simulink model "scen1_BSCproposed"  (R2021b)
settings: Solver=ode4  StartTime=0.0  StopTime=tsim  FixedStep=sampleRate  RelTol=1e-3
undefined symbols (not defined in the file): des_z, Kb, Kbz, peak_mp, Q, saturation_on, t_end_mp
libraries: dspmtrx3 x1
settings Model: Creator=PC  LastModifiedBy=kangm
settings SolverCC: AlgebraicLoopSolver=TrustRegion
settings DataIOCC: ReturnWorkspaceOutputs=off
settings DebuggingCC: SFMachineParentedDataDiag=warning

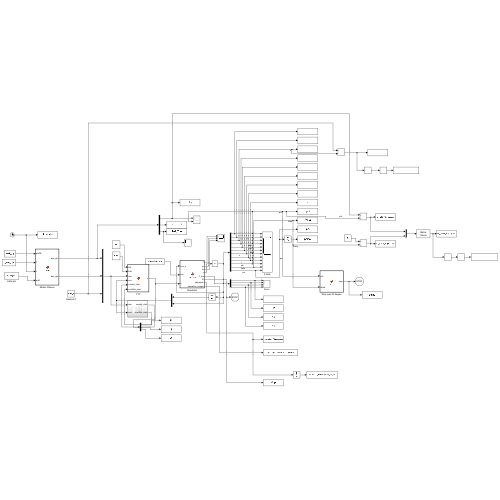
[thumbnail: Simulink's stored preview of the top-level diagram]
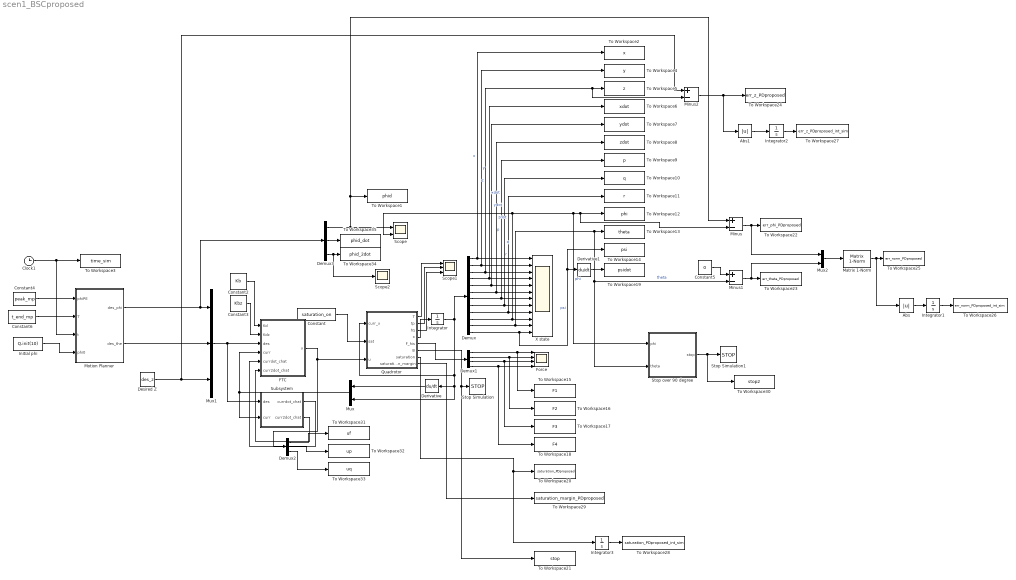
== system scen1_BSCproposed ==
  Abs : Abs
  Abs1 : Abs
  Clock1 : Clock
  Constant : Constant  Value=saturation_on
  Constant2 : Constant  Value=Kb
  Constant3 : Constant  Value=Kbz
  Constant4 : Constant  Value=peak_mp
  Constant5 : Constant  Value=0
  Constant6 : Constant  Value=t_end_mp
  Demux : Demux  Outputs=12
  Demux1 : Demux
  Demux2 : Demux  Outputs=3
  Demux3 : Demux  Outputs=3
  Derivative : Derivative
  Derivative1 : Derivative
  Desired Z : Constant  Value=des_z
  FTC : MATLAB Function  TreatAsAtomicUnit=on
  Force : Scope  NumInputPorts=4
  Initial phi : Constant  Value=Q.init(10)
  Integrator : Integrator  InitialCondition=Q.init
  Integrator1 : Integrator
  Integrator2 : Integrator
  Integrator3 : Integrator
  Matrix 1-Norm : dspmtrx3/Matrix  1-Norm  roundingMode=Floor  overflowMode=off  outputDataTypeStr=Inherit: Same as accumulator  outputMin=[]  outputMax=[]  outputLastDataTypeStr=Inherit: Same as accumulator
      settings: SourceProductBaseCode=DS
  Minus : Sum  Inputs=+-
  Minus1 : Sum  Inputs=+-
  Minus2 : Sum  Inputs=+-
  Motion Planner : MATLAB Function  TreatAsAtomicUnit=on
  Mux : Mux  Inputs=2
  Mux1 : Mux  Inputs=3
  Mux2 : Mux  Inputs=2
  Quadrotor : MATLAB Function  TreatAsAtomicUnit=on
  Scope : Scope  NumInputPorts=2
  Scope1 : Scope  NumInputPorts=3
  Scope2 : Scope
  Stop Simulation : Stop
  Stop Simulation1 : Stop
  Stop over 90 degree : MATLAB Function  TreatAsAtomicUnit=on
  Subsystem : Subsystem
  To Workspace1 : ToWorkspace  VariableName=phid  SampleTime=-1
      settings: Save2DSignal=2-D array (concatenate along first dimension)
  To Workspace10 : ToWorkspace  VariableName=q  SampleTime=-1
      settings: Save2DSignal=2-D array (concatenate along first dimension)
  To Workspace11 : ToWorkspace  VariableName=r  SampleTime=-1
      settings: Save2DSignal=2-D array (concatenate along first dimension)
  To Workspace12 : ToWorkspace  VariableName=phi  SampleTime=-1
      settings: Save2DSignal=2-D array (concatenate along first dimension)
  To Workspace13 : ToWorkspace  VariableName=theta  SampleTime=-1
      settings: Save2DSignal=2-D array (concatenate along first dimension)
  To Workspace14 : ToWorkspace  VariableName=psi  SampleTime=-1
      settings: Save2DSignal=2-D array (concatenate along first dimension)
  To Workspace15 : ToWorkspace  VariableName=F1  SampleTime=-1
      settings: Save2DSignal=2-D array (concatenate along first dimension)
  To Workspace16 : ToWorkspace  VariableName=F2  SampleTime=-1
      settings: Save2DSignal=2-D array (concatenate along first dimension)
  To Workspace17 : ToWorkspace  VariableName=F3  SampleTime=-1
      settings: Save2DSignal=2-D array (concatenate along first dimension)
  To Workspace18 : ToWorkspace  VariableName=F4  SampleTime=-1
      settings: Save2DSignal=2-D array (concatenate along first dimension)
  To Workspace19 : ToWorkspace  VariableName=psidot  SampleTime=-1
      settings: Save2DSignal=2-D array (concatenate along first dimension)
  To Workspace2 : ToWorkspace  VariableName=x  SampleTime=-1
      settings: Save2DSignal=2-D array (concatenate along first dimension)
  To Workspace20 : ToWorkspace  VariableName=saturation_PDproposed  SampleTime=-1
      settings: Save2DSignal=2-D array (concatenate along first dimension)
  To Workspace21 : ToWorkspace  VariableName=stop  SampleTime=-1
      settings: Save2DSignal=2-D array (concatenate along first dimension)
  To Workspace22 : ToWorkspace  VariableName=err_phi_PDproposed  SampleTime=-1
      settings: Save2DSignal=2-D array (concatenate along first dimension)
  To Workspace23 : ToWorkspace  VariableName=err_theta_PDproposed  SampleTime=-1
      settings: Save2DSignal=2-D array (concatenate along first dimension)
  To Workspace24 : ToWorkspace  VariableName=err_z_PDproposed  SampleTime=-1
      settings: Save2DSignal=2-D array (concatenate along first dimension)
  To Workspace25 : ToWorkspace  VariableName=err_norm_PDproposed  SampleTime=-1
      settings: Save2DSignal=2-D array (concatenate along first dimension)
  To Workspace26 : ToWorkspace  VariableName=err_norm_PDproposed_int_sim  SampleTime=-1
      settings: Save2DSignal=2-D array (concatenate along first dimension)
  To Workspace27 : ToWorkspace  VariableName=err_z_PDproposed_int_sim  SampleTime=-1
      settings: Save2DSignal=2-D array (concatenate along first dimension)
  To Workspace28 : ToWorkspace  VariableName=saturation_PDproposed_int_sim  SampleTime=-1
      settings: Save2DSignal=2-D array (concatenate along first dimension)
  To Workspace29 : ToWorkspace  VariableName=saturation_margin_PDproposed  SampleTime=-1
      settings: Save2DSignal=2-D array (concatenate along first dimension)
  To Workspace3 : ToWorkspace  VariableName=time_sim  SampleTime=-1
      settings: Save2DSignal=2-D array (concatenate along first dimension)
  To Workspace30 : ToWorkspace  VariableName=stop2  SampleTime=-1
      settings: Save2DSignal=2-D array (concatenate along first dimension)
  To Workspace31 : ToWorkspace  VariableName=uf  SampleTime=-1
      settings: Save2DSignal=2-D array (concatenate along first dimension)
  To Workspace32 : ToWorkspace  VariableName=up  SampleTime=-1
      settings: Save2DSignal=2-D array (concatenate along first dimension)
  To Workspace33 : ToWorkspace  VariableName=uq  SampleTime=-1
      settings: Save2DSignal=2-D array (concatenate along first dimension)
  To Workspace34 : ToWorkspace  VariableName=phid_2dot  SampleTime=-1
      settings: Save2DSignal=2-D array (concatenate along first dimension)
  To Workspace35 : ToWorkspace  VariableName=phid_dot  SampleTime=-1
      settings: Save2DSignal=2-D array (concatenate along first dimension)
  To Workspace4 : ToWorkspace  VariableName=y  SampleTime=-1
      settings: Save2DSignal=2-D array (concatenate along first dimension)
  To Workspace5 : ToWorkspace  VariableName=z  SampleTime=-1
      settings: Save2DSignal=2-D array (concatenate along first dimension)
  To Workspace6 : ToWorkspace  VariableName=xdot  SampleTime=-1
      settings: Save2DSignal=2-D array (concatenate along first dimension)
  To Workspace7 : ToWorkspace  VariableName=ydot  SampleTime=-1
      settings: Save2DSignal=2-D array (concatenate along first dimension)
  To Workspace8 : ToWorkspace  VariableName=zdot  SampleTime=-1
      settings: Save2DSignal=2-D array (concatenate along first dimension)
  To Workspace9 : ToWorkspace  VariableName=p  SampleTime=-1
      settings: Save2DSignal=2-D array (concatenate along first dimension)
  X state : Scope  NumInputPorts=12
  wires:
  Quadrotor/4(x) -> Integrator/1
  Mux1/1 -> Subsystem/1(des), FTC/3(des)
  Integrator/1 -> Quadrotor/1(curr_x), Derivative/1, Mux/2, Demux/1
  Demux/1 -> To Workspace2/1, X state/1  "x"
  Demux/2 -> To Workspace4/1, X state/2  "y"
  Demux/4 -> To Workspace6/1, X state/4  "xdot"
  Demux/5 -> To Workspace7/1, X state/5  "ydot"
  Demux/6 -> To Workspace8/1, X state/6  "zdot"
  Demux/7 -> To Workspace9/1, X state/7  "p"
  Demux/8 -> To Workspace10/1, X state/8  "q"
  Demux/9 -> To Workspace11/1, X state/9  "r"
  Mux/1 -> FTC/4(curr), Subsystem/2(curr)
  Derivative/1 -> Mux/1
  Quadrotor/5(F_his) -> Demux1/1
  Demux1/1 -> To Workspace15/1, Force/1
  Demux1/3 -> To Workspace17/1, Force/3
  Demux1/4 -> To Workspace18/1, Force/4
  Demux1/2 -> Force/2, To Workspace16/1
  Demux/12 -> To Workspace14/1, Derivative1/1, X state/12  "psi"
  Derivative1/1 -> To Workspace19/1
  Demux3/1 -> To Workspace1/1, Minus/1, Scope/1
  Constant/1 -> Quadrotor/2(sat)
  Clock1/1 -> Motion Planner/3(t), To Workspace3/1
  Initial phi/1 -> Motion Planner/4(phi0)
  Demux3/2 -> To Workspace35/1
  Demux3/3 -> Scope2/1, To Workspace34/1
  FTC/1(u) -> Demux2/1, Quadrotor/3(u)
  Quadrotor/1(T) -> Scope1/1
  Quadrotor/3(tq) -> Scope1/3
  Quadrotor/2(tp) -> Scope1/2
  Motion Planner/1(des_phi) -> Demux3/1, Mux1/1
  Motion Planner/2(des_the) -> Mux1/2
  Quadrotor/6(B) -> To Workspace21/1, Stop Simulation/1
  Desired Z/1 -> Minus2/1, Mux1/3
  Minus1/1 -> Mux2/2, To Workspace23/1
  Minus/1 -> Mux2/1, To Workspace22/1
  Demux/3 -> Minus2/2, To Workspace5/1, X state/3  "z"
  Mux2/1 -> Matrix 1-Norm/1
  Constant5/1 -> Minus1/1
  Integrator1/1 -> To Workspace26/1
  Matrix 1-Norm/1 -> Abs/1, To Workspace25/1
  Abs/1 -> Integrator1/1
  Constant4/1 -> Motion Planner/1(phiPE)
  Constant6/1 -> Motion Planner/2(T)
  Integrator2/1 -> To Workspace27/1
  Minus2/1 -> Abs1/1, To Workspace24/1
  Abs1/1 -> Integrator2/1
  Integrator3/1 -> To Workspace28/1
  Quadrotor/7(saturation) -> Integrator3/1, To Workspace20/1
  Quadrotor/8(saturation_margin) -> To Workspace29/1
  Demux/10 -> Scope/2, Stop over 90 degree/1(phi), Minus/2, To Workspace12/1, X state/10  "phi"
  Stop over 90 degree/1(stop) -> To Workspace30/1, Stop Simulation1/1
  Demux/11 -> Stop over 90 degree/2(theta), Minus1/2, To Workspace13/1, X state/11  "theta"
  Demux2/1 -> To Workspace31/1
  Demux2/2 -> To Workspace32/1
  Demux2/3 -> To Workspace33/1
  Constant2/1 -> FTC/1(Kd)
  Subsystem/1(currdot_chat) -> FTC/5(currdot_chat)
  Subsystem/2(curr2dot_chat) -> FTC/6(curr2dot_chat)
  Constant3/1 -> FTC/2(Kdz)

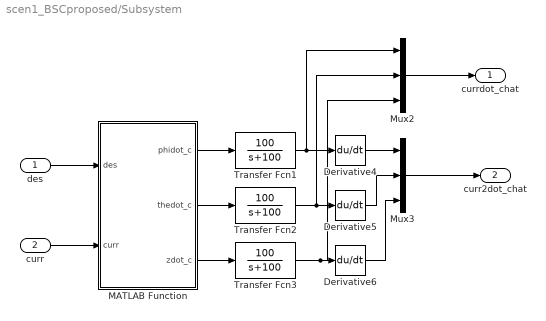
== system scen1_BSCproposed/Subsystem ==
  des : Inport
  curr : Inport  Port=2
  Derivative4 : Derivative
  Derivative5 : Derivative
  Derivative6 : Derivative
  MATLAB Function : MATLAB Function  TreatAsAtomicUnit=on
  Mux2 : Mux  Inputs=3
  Mux3 : Mux  Inputs=3
  Transfer Fcn1 : TransferFcn  Numerator=[100]  Denominator=[1 100]
  Transfer Fcn2 : TransferFcn  Numerator=[100]  Denominator=[1 100]
  Transfer Fcn3 : TransferFcn  Numerator=[100]  Denominator=[1 100]
  currdot_chat : Outport
  curr2dot_chat : Outport  Port=2
  wires:
  Derivative6/1 -> Mux3/3
  des/1 -> MATLAB Function/1(des)
  MATLAB Function/3(zdot_c) -> Transfer Fcn3/1
  Transfer Fcn2/1 -> Mux2/2, Derivative5/1
  MATLAB Function/1(phidot_c) -> Transfer Fcn1/1
  MATLAB Function/2(thedot_c) -> Transfer Fcn2/1
  Transfer Fcn3/1 -> Mux2/3, Derivative6/1
  Derivative4/1 -> Mux3/1
  Derivative5/1 -> Mux3/2
  Transfer Fcn1/1 -> Mux2/1, Derivative4/1
  Mux2/1 -> currdot_chat/1
  Mux3/1 -> curr2dot_chat/1
  curr/1 -> MATLAB Function/2(curr)

== matlab function scen1_BSCproposed/Quadrotor ==
  data: T output; tp output; tq output; curr_x input; sat input; u input; x output; F_his output; B output; saturation output; saturation_margin output
function [T,tp,tq,x,F_his,B,saturation,saturation_margin] = system(curr_x,sat,u)
% x = {xyz xyzvel pqr phi theta psi}
x = zeros(12,1);
% Properties
m = 1.282; g = 9.81;
Ix = 4.856*10^-3; Iz = 8.801*10^-3;
b = 0.0066;
kr = 0.02; %drag coefficient
kt = 0.5;
l = 0.1;

u_temp = zeros(3,1);
u_temp = u;
u = u_temp;

T = u(1); tp = u(2); tq = u(3);% tr = u(4);
tr = b*(T-2*tp/l);
A = [1 1 1; 0 l 0;-l 0 l];

F=inv(A)*[T tp tq]';

f1 = F(1); f2 = F(2); f3 = F(3);
ub = 8.38;
lb = 0;

saturation1_lb = 0;
saturation1_ub = 0;
saturation2_lb = 0;
saturation2_ub = 0;
saturation3_lb = 0;
saturation3_ub = 0;
saturation1_lb_margin = 0;
saturation1_ub_margin = 0;
saturation2_lb_margin = 0;
saturation2_ub_margin = 0;
saturation3_lb_margin = 0;
saturation3_ub_margin = 0;

if sat == 1
    if f1 < lb
        saturation1_lb = abs(lb - f1);
        saturation1_lb_margin = abs(lb - f1);
        f1 = lb;
    else
        saturation1_lb_margin = lb - f1;
    end
    
    if f1 > ub
        saturation1_ub = abs(ub - f1);
        saturation1_ub_margin = abs(ub - f1);
        f1 = ub;
    else
        saturation1_ub_margin = f1 - ub;
    end
    
    if f2 < lb
        saturation2_lb = abs(lb - f2);
        saturation2_lb_margin = abs(lb - f2);
        f2 = lb;
    else
        saturation2_lb_margin = lb - f2;
    end
    
    if f2 > ub
        saturation2_ub = abs(ub - f2);
        saturation2_ub_margin = abs(ub - f2);
        f2 = ub;
    else
        saturation2_ub_margin = f2 - ub;
    end
    
    if f3 < lb
        saturation3_lb = abs(lb - f3);
        saturation3_lb_margin = abs(lb - f3);
        f3 = lb;
    else
        saturation3_lb_margin = lb - f3;
    end
    
    if f3 > ub
        saturation3_ub = abs(ub - f3);
        saturation3_ub_margin = abs(ub - f3);
        f3 = ub;
    else
        saturation3_ub_margin = f3 - ub;
    end
end

saturation = max([saturation1_lb,saturation1_ub,saturation2_lb,saturation2_ub,saturation3_lb,saturation3_ub]);
saturation_margin = max([saturation1_lb_margin,saturation1_ub_margin,saturation2_lb_margin,saturation2_ub_margin,saturation3_lb_margin,saturation3_ub_margin]);

f4 = 0;
F_his = [f1 f2 f3 f4]';
T = f1+f2+f3;
tp = l*(f2);
tq = l*(f3-f1);
tr = b*(f1+f3-f2);


% Current state
x1  = curr_x(1);
x2  = curr_x(2);
x3  = curr_x(3);
x4  = curr_x(4);
x5  = curr_x(5);
x6  = curr_x(6);
x7  = curr_x(7);
x8  = curr_x(8);
x9  = curr_x(9);
x10 = curr_x(10);
x11 = curr_x(11);
x12 = curr_x(12);


% Position
x(1) = x4;
x(2) = x5;
x(3) = x6;
% Velocity
x(4) = T/m*(cos(x12)*sin(x11)*cos(x10) + sin(x12)*sin(x10)) - kt/m*x4;
x(5) = T/m*(sin(x12)*sin(x11)*cos(x10) - cos(x12)*sin(x10)) - kt/m*x5;
x(6) = -g + T*(1/m)*(cos(x10)*cos(x11)) - kt/m*x6;
% Body rate
x(7) = ((Ix-Iz)*x8*x9 + tp)/Ix;
x(8) = ((Iz-Ix)*x7*x9 + tq)/Ix;
x(9) = (-kr*x9 + tr)/Iz;
% Angle
x(10) = x7 + x8*sin(x10)*tan(x11) + x9*cos(x10)*tan(x11);
x(11) = x8*cos(x10) - x9*sin(x10);
x(12) = x8*sin(x10)/cos(x11) + x9*cos(x10)*cos(x11);

if x3<=0
    B=1;
else
    B=0;
end

% x;
% 
% r_c = 10.2020-2.2725*x9;
% u_c = (x(7)-((Ix-Iz)/Ix)*x8*x9)*Ix+x10;
% r_ct = -4.489*exp(-2.2725*t)+4.489;

== matlab function scen1_BSCproposed/Stop over 90 degree ==
  data: phi input; stop output; theta input
function stop = fcn(phi, theta)

stop = 0;
max_attitude = deg2rad(90);

if abs(phi) >= max_attitude || abs(theta) >= max_attitude
    stop = 1;
end

== matlab function scen1_BSCproposed/Motion Planner ==
  data: phiPE input; T input; des_phi output; des_the output; t input; phi0 input
function [des_phi,des_the]  = fcn(phiPE,T,t,phi0)


% b = deg2rad(20); % Periodic solution phi
% t_end = 5;
a0 = phi0;
a1 = 0;
a2 = 0;
a3 = - (10*phi0 - 10*phiPE)/T^3;
a4 = (15*phi0 - 15*phiPE)/T^4;
a5 = -(6*phi0 - 6*phiPE)/T^5;

if t <= T
    phi_d = a0 + a1*t + a2*t^2 + a3*t^3 + a4*t^4 + a5*t^5; % phi_d(0) = phi(0) and phi_d(t_end) = phi hat (periodic solution)
    phidot_d = a1 + 2*a2*t + 3*a3*t^2 + 4*a4*t^3 + 5*a5*t^4; % phidot_d(t_end) = 0
    phi2dot_d = 2*a2 + 6*a3*t + 12*a4*t^2 + 20*a5*t^3;
else
    phi_d = phiPE;
    phidot_d = 0;
    phi2dot_d = 0;
end

% phidot_d = 0;

the_d = deg2rad(0); thedot_d = 0; the2dot_d = 0;


des_phi = [phi_d, phidot_d, phi2dot_d]';
des_the = [the_d, thedot_d, the2dot_d]';

== matlab function scen1_BSCproposed/FTC ==
  data: Kd input; Kdz input; des input; u output; curr input; currdot_chat input; curr2dot_chat input
function u   = bsc(Kd,Kdz,des,curr,currdot_chat,curr2dot_chat)

m = 1.282; g = 9.81;
Ix = 4.856*10^-3; Iy = Ix; Iz = 8.801*10^-3;
b = 0.0066;
kr = 0.02; %drag coefficient
kt = 0.5;
% kt = 0.25;
l = 0.1;

% current state
N = 0;
xdot   = curr(N+1); ydot   = curr(N+2); zdot   = curr(N+3);
x2dot  = curr(N+4); y2dot  = curr(N+5); z2dot  = curr(N+6);
pdot   = curr(N+7); qdot   = curr(N+8); rdot   = curr(N+9);
phidot = curr(N+10);thedot = curr(N+11);psidot = curr(N+12);

N = 12;
x    = curr(N+1); y    = curr(N+2); z    = curr(N+3);
xdot = curr(N+4); ydot = curr(N+5); zdot = curr(N+6);
p    = curr(N+7); q    = curr(N+8); r    = curr(N+9);
phi  = curr(N+10);the  = curr(N+11);psi  = curr(N+12);
des_temp = zeros(7,1);
des_temp = des;
des = des_temp;
% desired state
phi_d = des(1);
phidot_d = des(2);
phi2dot_d = des(3);
the_d = des(4);
thedot_d = des(5);
the2dot_d = des(6);
z_d   = des(7);

phidot_chat = currdot_chat(1);
thedot_chat = currdot_chat(2);
zdot_chat = currdot_chat(3);
phi2dot_chat = curr2dot_chat(1);
the2dot_chat = curr2dot_chat(2);
z2dot_chat = curr2dot_chat(3);

F = [p + q*sin(phi)*tan(the) + r*cos(phi)*tan(the)
     q*cos(phi) - r*sin(phi)
     -(Iz - Iy)*q*r/Ix
     -(Ix - Iz)*p*r/Iy
     -kr*r/Iz
     zdot
     -kt*zdot/m - g];
 
G = [0 0 0
     0 0 0
     0 1/Ix 0
     0 0 1/Iy
     b/Iz -2*b/(l*Iz) 0
     0 0 0
     cos(phi)*cos(the)/m 0 0];
 
J = [q*cos(phi)*tan(the)-r*sin(phi)*tan(the) q*sin(phi)*sec(the)^2+r*cos(phi)*sec(the)^2 1 sin(phi)*tan(the) cos(phi)*tan(the) 0 0
     -q*sin(phi)-r*cos(phi) 0 0 cos(phi) -sin(phi) 0 0
     0 0 0 0 0 0 1];

ubar = [phi2dot_chat + (phi_d-phi) + Kd*(phidot_chat-phidot)
        the2dot_chat + (the_d-the) + Kd*(thedot_chat-thedot)
        z2dot_chat + (0-zdot) + Kdz*(zdot_chat-zdot)];
    
u = inv(J*G)*(-J*F + ubar);

== matlab function scen1_BSCproposed/Subsystem/MATLAB Function ==
  data: des input; phidot_c output; curr input; thedot_c output; zdot_c output
function [phidot_c,thedot_c,zdot_c] = fcn(des, curr)

% current state
N = 0;
xdot   = curr(N+1); ydot   = curr(N+2); zdot   = curr(N+3);
x2dot  = curr(N+4); y2dot  = curr(N+5); z2dot  = curr(N+6);
pdot   = curr(N+7); qdot   = curr(N+8); rdot   = curr(N+9);
phidot = curr(N+10);thedot = curr(N+11);psidot = curr(N+12);

N = 12;
x    = curr(N+1); y    = curr(N+2); z    = curr(N+3);
xdot = curr(N+4); ydot = curr(N+5); zdot = curr(N+6);
p    = curr(N+7); q    = curr(N+8); r    = curr(N+9);
phi  = curr(N+10);the  = curr(N+11);psi  = curr(N+12);

% desired state
phi_d = des(1);
phidot_d = des(2);
phi2dot_d = des(3);
the_d = des(4);
thedot_d = des(5);
the2dot_d = des(6);
z_d   = des(7);
zdot_d = 0;

K = 22;

phidot_c = phidot_d + K*(phi_d-phi);
thedot_c = thedot_d + K*(the_d-the);
zdot_c = zdot_d + K*(z_d-z);
